simulink model "EsamblajeCohete2_0"  (R2022a)
settings: Solver=VariableStepAuto  StartTime=0.0  StopTime=10.0  RelTol=1e-3
model workspace: external: MATLAB File C:\Users\SEBASTIANDIAZPABON\OneDrive - Universidad Santo Tomás Bucaramanga\USTA\Semillero Cohete\Cohete Matlab 2.0\EsamblajeCohete2_0_DataFile.m (data not in the file)
undefined symbols (not defined in the file or in its folder): smiData, X, Y, Z
libraries: sm_lib x340, simulink x39, nesl_utility x9
(part 4 of 6)

== system EsamblajeCohete2_0/Cohete/x13_INCH_PROPELLER_2_RIGID ==
  ReferenceFrame : sm_lib/Frames and Transforms/Reference Frame
  Solid : sm_lib/Body Elements/File Solid  ExtGeomFileName=13 INCH PROPELLER_Default_sldprt.STEP  UnitType=FromFile  ExtGeomFileUnits=m  StepReaderType=HEX  ExportConvexHullGeometry=off  InertiaType=Custom  Mass=smiData.Solid(1).mass  MassUnits=kg  CenterOfMass=smiData.Solid(1).CoM  CenterOfMassUnits=mm  MomentsOfInertia=smiData.Solid(1).MoI  MomentsOfInertiaUnits=kg*mm^2  ProductsOfInertia=smiData.Solid(1).PoI  ProductsOfInertiaUnits=kg*mm^2  BasedOnType=DensityFromFile  Density=1000  DensityUnits=kg/m^3  DoExposeReferenceFrame=on  SerializedFrames=<Frames/>  GraphicType=FromGeometry  MarkerShape=Sphere  MarkerSize=10  GraphicVisPropType=SimpleVisualProperties  GraphicDiffuseColor=smiData.Solid(1).color  GraphicSpecularColor=[0.5 0.5 0.5 1.0]  GraphicAmbientColor=[0.15 0.15 0.15 1.0]  GraphicEmissiveColor=[0.0 0.0 0.0 1.0]  GraphicShininess=75  GraphicOpacity=smiData.Solid(1).opacity
  Transform : sm_lib/Frames and Transforms/Rigid Transform  TranslationMethod=Cartesian  TranslationStandardOffset=0  TranslationLengthUnit=mm  TranslationStandardAxis=+Z  TranslationCartesianOffset=smiData.RigidTransform(4).translation  TranslationROffset=0  TranslationROffsetUnits=m  TranslationZOffset=0  TranslationZOffsetUnits=m  TranslationThetaOffset=0  TranslationThetaOffsetUnits=deg  RotationMethod=ArbitraryAxis  RotationAngleUnits=rad  RotationStandardAxis=+Z  RotationAngle=smiData.RigidTransform(4).angle  RotationArbitraryAxis=smiData.RigidTransform(4).axis  FollAlignAxisA=+X  BaseAlignAxisA=+Y  FollAlignAxisB=+Y  BaseAlignAxisB=+Z  RotationSequenceAxes=FollowerAxes  RotationSequence=XYX  RotationSequenceAngles=[0 0 0]  RotationSequenceAnglesUnits=deg  RotationMatrix=[1 0 0; 0 1 0; 0 0 1]
  F : PMIOPort  Side=Left
  connections:
  Solid/RConn1 -- ReferenceFrame/RConn1 -- Transform/LConn1
  Transform/RConn1 -- F/RConn1

== system EsamblajeCohete2_0/Cohete/x13_INCH_PROPELLER_3_RIGID ==
  ReferenceFrame : sm_lib/Frames and Transforms/Reference Frame
  Solid : sm_lib/Body Elements/File Solid  ExtGeomFileName=13 INCH PROPELLER_Default_sldprt.STEP  UnitType=FromFile  ExtGeomFileUnits=m  StepReaderType=HEX  ExportConvexHullGeometry=off  InertiaType=Custom  Mass=smiData.Solid(1).mass  MassUnits=kg  CenterOfMass=smiData.Solid(1).CoM  CenterOfMassUnits=mm  MomentsOfInertia=smiData.Solid(1).MoI  MomentsOfInertiaUnits=kg*mm^2  ProductsOfInertia=smiData.Solid(1).PoI  ProductsOfInertiaUnits=kg*mm^2  BasedOnType=DensityFromFile  Density=1000  DensityUnits=kg/m^3  DoExposeReferenceFrame=on  SerializedFrames=<Frames/>  GraphicType=FromGeometry  MarkerShape=Sphere  MarkerSize=10  GraphicVisPropType=SimpleVisualProperties  GraphicDiffuseColor=smiData.Solid(1).color  GraphicSpecularColor=[0.5 0.5 0.5 1.0]  GraphicAmbientColor=[0.15 0.15 0.15 1.0]  GraphicEmissiveColor=[0.0 0.0 0.0 1.0]  GraphicShininess=75  GraphicOpacity=smiData.Solid(1).opacity
  Transform : sm_lib/Frames and Transforms/Rigid Transform  TranslationMethod=Cartesian  TranslationStandardOffset=0  TranslationLengthUnit=mm  TranslationStandardAxis=+Z  TranslationCartesianOffset=smiData.RigidTransform(6).translation  TranslationROffset=0  TranslationROffsetUnits=m  TranslationZOffset=0  TranslationZOffsetUnits=m  TranslationThetaOffset=0  TranslationThetaOffsetUnits=deg  RotationMethod=ArbitraryAxis  RotationAngleUnits=rad  RotationStandardAxis=+Z  RotationAngle=smiData.RigidTransform(6).angle  RotationArbitraryAxis=smiData.RigidTransform(6).axis  FollAlignAxisA=+X  BaseAlignAxisA=+Y  FollAlignAxisB=+Y  BaseAlignAxisB=+Z  RotationSequenceAxes=FollowerAxes  RotationSequence=XYX  RotationSequenceAngles=[0 0 0]  RotationSequenceAnglesUnits=deg  RotationMatrix=[1 0 0; 0 1 0; 0 0 1]
  F : PMIOPort  Side=Left
  connections:
  Solid/RConn1 -- ReferenceFrame/RConn1 -- Transform/LConn1
  Transform/RConn1 -- F/RConn1

== system EsamblajeCohete2_0/Cohete/x13_INCH_PROPELLER_4_RIGID ==
  ReferenceFrame : sm_lib/Frames and Transforms/Reference Frame
  Solid : sm_lib/Body Elements/File Solid  ExtGeomFileName=13 INCH PROPELLER_Default_sldprt.STEP  UnitType=FromFile  ExtGeomFileUnits=m  StepReaderType=HEX  ExportConvexHullGeometry=off  InertiaType=Custom  Mass=smiData.Solid(1).mass  MassUnits=kg  CenterOfMass=smiData.Solid(1).CoM  CenterOfMassUnits=mm  MomentsOfInertia=smiData.Solid(1).MoI  MomentsOfInertiaUnits=kg*mm^2  ProductsOfInertia=smiData.Solid(1).PoI  ProductsOfInertiaUnits=kg*mm^2  BasedOnType=DensityFromFile  Density=1000  DensityUnits=kg/m^3  DoExposeReferenceFrame=on  SerializedFrames=<Frames/>  GraphicType=FromGeometry  MarkerShape=Sphere  MarkerSize=10  GraphicVisPropType=SimpleVisualProperties  GraphicDiffuseColor=smiData.Solid(1).color  GraphicSpecularColor=[0.5 0.5 0.5 1.0]  GraphicAmbientColor=[0.15 0.15 0.15 1.0]  GraphicEmissiveColor=[0.0 0.0 0.0 1.0]  GraphicShininess=75  GraphicOpacity=smiData.Solid(1).opacity
  Transform : sm_lib/Frames and Transforms/Rigid Transform  TranslationMethod=Cartesian  TranslationStandardOffset=0  TranslationLengthUnit=mm  TranslationStandardAxis=+Z  TranslationCartesianOffset=smiData.RigidTransform(8).translation  TranslationROffset=0  TranslationROffsetUnits=m  TranslationZOffset=0  TranslationZOffsetUnits=m  TranslationThetaOffset=0  TranslationThetaOffsetUnits=deg  RotationMethod=ArbitraryAxis  RotationAngleUnits=rad  RotationStandardAxis=+Z  RotationAngle=smiData.RigidTransform(8).angle  RotationArbitraryAxis=smiData.RigidTransform(8).axis  FollAlignAxisA=+X  BaseAlignAxisA=+Y  FollAlignAxisB=+Y  BaseAlignAxisB=+Z  RotationSequenceAxes=FollowerAxes  RotationSequence=XYX  RotationSequenceAngles=[0 0 0]  RotationSequenceAnglesUnits=deg  RotationMatrix=[1 0 0; 0 1 0; 0 0 1]
  F : PMIOPort  Side=Left
  connections:
  Solid/RConn1 -- ReferenceFrame/RConn1 -- Transform/LConn1
  Transform/RConn1 -- F/RConn1

== system EsamblajeCohete2_0/Dinámica /Constantes ==
  Masa : Constant  Value=1.6
  gravedad : Constant  Value=9.81
  ixx : Constant  Value=0.04
  ixx1 : Constant  Value=0.04
  iyy : Constant  Value=0.02
  kd : Constant
  kt : Constant
  longitud : Constant  Value=0.2923
  m : Outport
  g : Outport  Port=2
  Ixx : Outport  Port=3
  Iyy : Outport  Port=4
  Izz : Outport  Port=5
  L : Outport  Port=6
  Κτ : Outport  Port=7
  Kd : Outport  Port=8
  wires:
  Masa/1 -> m/1
  gravedad/1 -> g/1
  ixx/1 -> Ixx/1
  iyy/1 -> Iyy/1
  ixx1/1 -> Izz/1
  longitud/1 -> L/1
  kt/1 -> Κτ/1
  kd/1 -> Kd/1

== system EsamblajeCohete2_0/Dinámica /Torque Yaw ==
  note: $\tau_\psi=\sum_{i=1}^4 \tau_{M i}=K_d \cdot\left(-\omega_1^2+\omega_2^2-\omega_3^2+\omega_4^2\right)$
  ω1 : Inport
  ω2 : Inport  Port=2
  ω3 : Inport  Port=3
  ω4 : Inport  Port=4
  Kd : Inport  Port=5
  Add : Sum  Inputs=-+-+
  Dot Product{,1..7} (8 alike) : DotProduct  OutDataTypeStr=Inherit: Inherit via internal rule
  Tψ : Outport
  wires:
  ω1/1 -> Dot Product/1, Dot Product/2
  Dot Product1/1 -> Add/1
  Dot Product/1 -> Dot Product1/2
  Kd/1 -> Dot Product7/1, Dot Product5/1, Dot Product3/1, Dot Product1/1
  ω2/1 -> Dot Product2/2, Dot Product2/1
  Dot Product2/1 -> Dot Product3/2
  Dot Product3/1 -> Add/2
  ω3/1 -> Dot Product4/2, Dot Product4/1
  Dot Product4/1 -> Dot Product5/2
  Dot Product5/1 -> Add/3
  ω4/1 -> Dot Product6/2, Dot Product6/1
  Dot Product6/1 -> Dot Product7/2
  Dot Product7/1 -> Add/4
  Add/1 -> Tψ/1

== system EsamblajeCohete2_0/Dinámica /Torques Roll y Pitch ==
  note: $\tau_\phi=l \cdot\left(f_4-f_2\right)$
  note: $\tau_\theta=l \cdot\left(f_3-f_1\right)$
  L : Inport
  f1 : Inport  Port=2
  f2 : Inport  Port=3
  f3 : Inport  Port=4
  f4 : Inport  Port=5
  Add : Sum  Inputs=+-
  Add1 : Sum  Inputs=+-
  Product{,1..3} (4 alike) : Product
  Tφ : Outport
  Tθ : Outport  Port=2
  wires:
  f1/1 -> Product/2
  L/1 -> Product1/1, Product3/1, Product2/1, Product/1
  f3/1 -> Product1/2
  Product1/1 -> Add/1
  Product/1 -> Add/2
  Add/1 -> Tθ/1
  f4/1 -> Product2/2
  f2/1 -> Product3/2
  Product2/1 -> Add1/1
  Product3/1 -> Add1/2
  Add1/1 -> Tφ/1

== system EsamblajeCohete2_0/Dinámica /Z'' ==
  note: $\ddot{z}=\frac{f}{m} cos( \phi) cos( \theta)-g$
  f : Inport
  m : Inport  Port=2
  g : Inport  Port=3
  ϕ : Inport  Port=4
  θ : Inport  Port=5
  Add : Sum  Inputs=+-
  Divide : Product  Inputs=*/
  Dot Product1 : DotProduct  OutDataTypeStr=Inherit: Inherit via internal rule
  Integrator : Integrator
  Integrator1 : Integrator
  Product2 : Product
  cos(θ) : simulink/Lookup Tables/Cosine  Formula=cos(2*pi*u)  NumDataPoints=(2^5)+1  OutputWordLength=16  InternalRulePriority=Speed
      settings: SourceProductBaseCode=SL
  cos(ϕ) : simulink/Lookup Tables/Cosine  Formula=cos(2*pi*u)  NumDataPoints=(2^5)+1  OutputWordLength=16  InternalRulePriority=Speed
      settings: SourceProductBaseCode=SL
  Z : Outport
  wires:
  g/1 -> Add/2
  f/1 -> Divide/1
  m/1 -> Divide/2
  Divide/1 -> Product2/1
  Product2/1 -> Add/1
  Integrator1/1 -> Z/1
  Integrator/1 -> Integrator1/1
  Add/1 -> Integrator/1
  θ/1 -> cos(θ)/1
  ϕ/1 -> cos(ϕ)/1
  cos(ϕ)/1 -> Dot Product1/1
  cos(θ)/1 -> Dot Product1/2
  Dot Product1/1 -> Product2/2

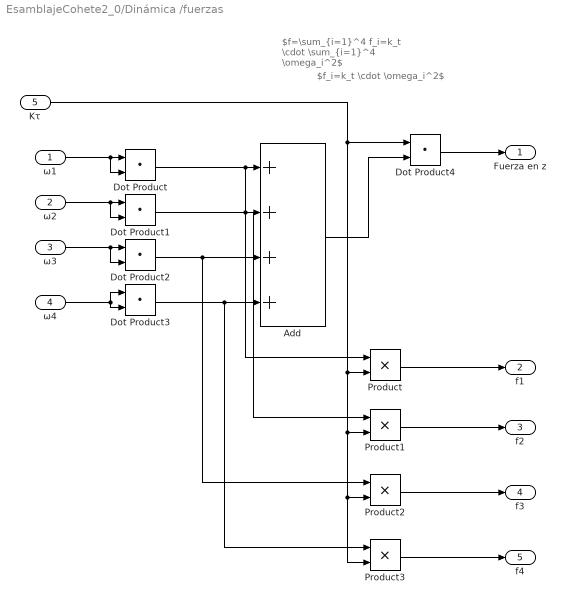
== system EsamblajeCohete2_0/Dinámica /fuerzas ==
  note: $f_i=k_t \cdot \omega_i^2$
  note: $f=\sum_{i=1}^4 f_i=k_t \cdot \sum_{i=1}^4 \omega_i^2$
  ω1 : Inport
  ω2 : Inport  Port=2
  ω3 : Inport  Port=3
  ω4 : Inport  Port=4
  Κτ : Inport  Port=5
  Add : Sum  Inputs=++++
  Dot Product{,1..4} (5 alike) : DotProduct  OutDataTypeStr=Inherit: Inherit via internal rule
  Product{,1..3} (4 alike) : Product
  Fuerza en z : Outport
  f1 : Outport  Port=2
  f2 : Outport  Port=3
  f3 : Outport  Port=4
  f4 : Outport  Port=5
  wires:
  ω1/1 -> Dot Product/2, Dot Product/1
  Dot Product/1 -> Product/1, Add/1
  ω2/1 -> Dot Product1/2, Dot Product1/1
  ω3/1 -> Dot Product2/2, Dot Product2/1
  ω4/1 -> Dot Product3/1, Dot Product3/2
  Dot Product1/1 -> Product1/1, Add/2
  Dot Product2/1 -> Product2/1, Add/3
  Dot Product3/1 -> Product3/1, Add/4
  Dot Product4/1 -> Fuerza en z/1
  Κτ/1 -> Product3/2, Product2/2, Product1/2, Product/2, Dot Product4/1
  Add/1 -> Dot Product4/2
  Product/1 -> f1/1
  Product1/1 -> f2/1
  Product2/1 -> f3/1
  Product3/1 -> f4/1

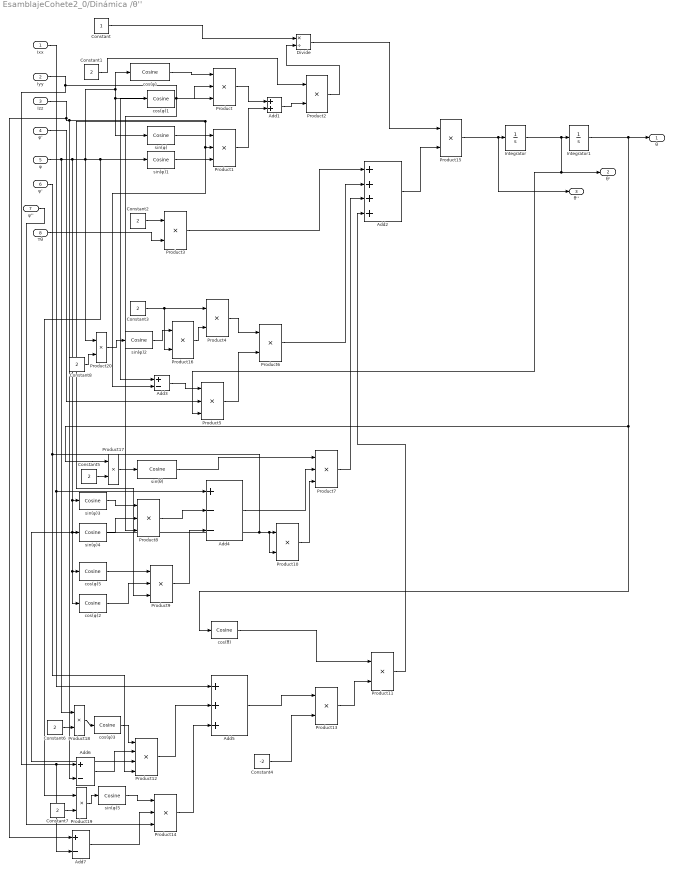
== system EsamblajeCohete2_0/Dinámica /θ'' ==
  Ixx : Inport
  Iyy : Inport  Port=2
  Izz : Inport  Port=3
  φ' : Inport  Port=4
  φ : Inport  Port=5
  ψ' : Inport  Port=6
  ψ'' : Inport  Port=7
  Tθ : Inport  Port=8
  Add1 : Sum
  Add2 : Sum  Inputs=++++
  Add3 : Sum  Inputs=+-
  Add4 : Sum  Inputs=+--
  Add5 : Sum  Inputs=+++
  Add6 : Sum  Inputs=+-
  Add7 : Sum  Inputs=+-
  Constant : Constant
  Constant{1..3,5..8} (7 alike) : Constant  Value=2
  Constant4 : Constant  Value=-2
  Divide : Product  Inputs=*/
  Integrator : Integrator
  Integrator1 : Integrator
  Product{,1,5,7..9,14} (7 alike) : Product  Inputs=3
  Product{2..4,6,10..11,13,15..20} (13 alike) : Product
  Product12 : Product  Inputs=4
  cos(θ) : simulink/Lookup Tables/Cosine  Formula=cos(2*pi*u)  NumDataPoints=(2^5)+1  OutputWordLength=16  InternalRulePriority=Speed
      settings: SourceProductBaseCode=SL
  cos(φ){,1..3,5} (5 alike) : simulink/Lookup Tables/Cosine  Formula=cos(2*pi*u)  NumDataPoints=(2^5)+1  OutputWordLength=16  InternalRulePriority=Speed
      settings: SourceProductBaseCode=SL
  sin(θ) : simulink/Lookup Tables/Cosine  Formula=sin(2*pi*u)  NumDataPoints=(2^5)+1  OutputWordLength=16  InternalRulePriority=Speed
      settings: SourceProductBaseCode=SL
  sin(φ){,1..5} (6 alike) : simulink/Lookup Tables/Cosine  Formula=sin(2*pi*u)  NumDataPoints=(2^5)+1  OutputWordLength=16  InternalRulePriority=Speed
      settings: SourceProductBaseCode=SL
  θ : Outport
  θ' : Outport  Port=2
  θ'' : Outport  Port=3
  wires:
  Constant/1 -> Divide/1
  φ/1 -> Product18/1, cos(φ)2/1, cos(φ)5/1, sin(φ)4/1, sin(φ)3/1, Product20/1, Product19/1, sin(φ)1/1, cos(φ)1/1, sin(φ)/1, cos(φ)/1
  cos(φ)/1 -> Product/1
  cos(φ)1/1 -> Product/2
  Iyy/1 -> Add7/2, Add6/1, Add3/1, Product/3, Product8/3
  sin(φ)/1 -> Product1/1
  sin(φ)1/1 -> Product1/3
  Izz/1 -> Add7/1, Add3/2, Product1/2, Product9/3, Add6/2
  Product/1 -> Add1/1
  Product1/1 -> Add1/2
  Add1/1 -> Product2/2
  Constant1/1 -> Product2/1
  Product2/1 -> Divide/2
  Constant2/1 -> Product3/1
  Tθ/1 -> Product3/2
  Product3/1 -> Add2/1
  Constant3/1 -> Product16/2, Product4/1
  sin(φ)2/1 -> Product16/1
  Add3/1 -> Product5/1
  φ'/1 -> Product5/2
  Product4/1 -> Product6/1
  Product5/1 -> Product6/2
  Product6/1 -> Add2/2
  sin(θ)/1 -> Product7/1
  Ixx/1 -> Add5/1, Add4/1
  sin(φ)4/1 -> Product8/2
  sin(φ)3/1 -> Product8/1
  Product8/1 -> Add4/2
  cos(φ)5/1 -> Product9/1
  cos(φ)2/1 -> Product9/2
  Product9/1 -> Add4/3
  Add4/1 -> Product7/2
  ψ'/1 -> Product12/4, Product12/3, Product10/2, Product10/1
  Product10/1 -> Product7/3
  cos(θ)/1 -> Product11/1
  cos(φ)3/1 -> Product12/1
  Add6/1 -> Product12/2
  Product12/1 -> Add5/2
  Constant4/1 -> Product13/2
  Add5/1 -> Product13/1
  Product13/1 -> Product11/2
  sin(φ)5/1 -> Product14/1
  Add7/1 -> Product14/2
  Product14/1 -> Add5/3
  ψ''/1 -> Product14/3
  Product7/1 -> Add2/3
  Product11/1 -> Add2/4
  Divide/1 -> Product15/1
  Add2/1 -> Product15/2
  Product15/1 -> θ''/1, Integrator/1
  Integrator/1 -> θ'/1, Product5/3, Integrator1/1
  Integrator1/1 -> Product17/1, cos(θ)/1, θ/1
  Product16/1 -> Product4/2
  Product17/1 -> sin(θ)/1
  Constant5/1 -> Product17/2
  Constant6/1 -> Product18/2
  Product18/1 -> cos(φ)3/1
  Constant7/1 -> Product19/2
  Product19/1 -> sin(φ)5/1
  Constant8/1 -> Product20/2
  Product20/1 -> sin(φ)2/1

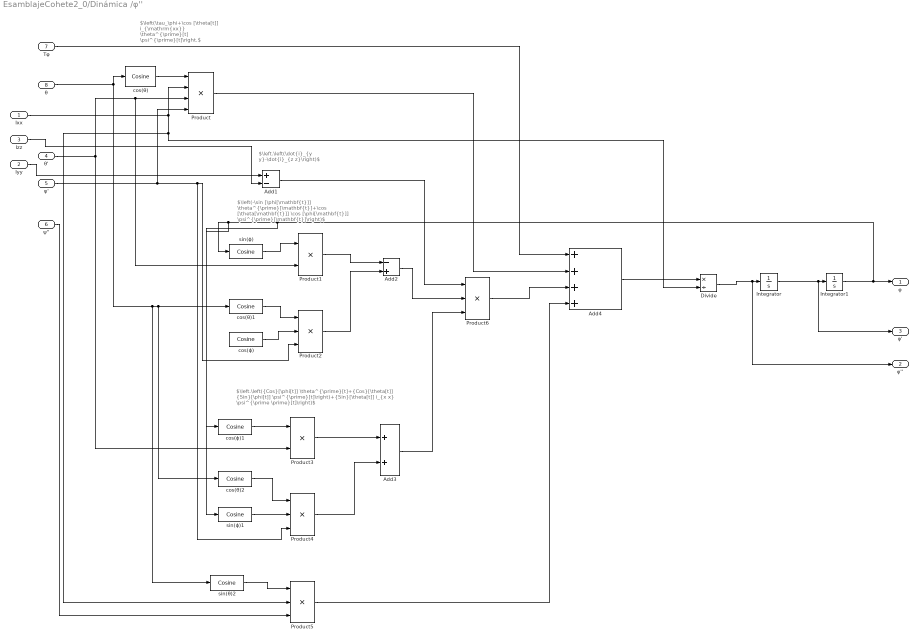
== system EsamblajeCohete2_0/Dinámica /φ'' ==
  note: $\left.\left({Cos}[\phi[t]] \theta^{\prime}[t]+{Cos}[\theta[t]] {Sin}[\phi[t]] \psi^{\prime}[t]\right)+{Sin}[\theta[t]] i_{x x} \psi^{\prime \prime}[t]\right)$
  note: $\left(-\sin [\phi[\mathbf{t}]] \theta^{\prime}[\mathbf{t}]+\cos [\theta[\mathbf{t}]] \cos [\phi[\mathbf{t}]] \psi^{\prime}[\mathbf{t}]\right)$
  note: $\left.\left(\dot{i}_{y y}-\dot{i}_{z z}\right)$
  note: $\left(\tau_\phi+\cos [\theta[t]] i_{\mathrm{xx}} \theta^{\prime}[t] \psi^{\prime}[t]\right.$
  Ixx : Inport
  Iyy : Inport  Port=2
  Izz : Inport  Port=3
  θ' : Inport  Port=4
  ψ' : Inport  Port=5
  ψ'' : Inport  Port=6
  Tφ : Inport  Port=7
  θ : Inport  Port=8
  Add1 : Sum  Inputs=+-
  Add2 : Sum  Inputs=-+
  Add3 : Sum
  Add4 : Sum  Inputs=++++
  Divide : Product  Inputs=*/
  Integrator : Integrator
  Integrator1 : Integrator
  Product : Product  Inputs=4
  Product1 : Product
  Product{2,4..6} (4 alike) : Product  Inputs=3
  Product3 : Product
  cos(θ) : simulink/Lookup Tables/Cosine  Formula=cos(2*pi*u)  NumDataPoints=(2^5)+1  OutputWordLength=16  InternalRulePriority=Speed
      settings: SourceProductBaseCode=SL
  cos(θ)1 : simulink/Lookup Tables/Cosine  Formula=cos(2*pi*u)  NumDataPoints=(2^5)+1  OutputWordLength=16  InternalRulePriority=Speed
      settings: SourceProductBaseCode=SL
  cos(θ)2 : simulink/Lookup Tables/Cosine  Formula=cos(2*pi*u)  NumDataPoints=(2^5)+1  OutputWordLength=16  InternalRulePriority=Speed
      settings: SourceProductBaseCode=SL
  cos(ϕ) : simulink/Lookup Tables/Cosine  Formula=cos(2*pi*u)  NumDataPoints=(2^5)+1  OutputWordLength=16  InternalRulePriority=Speed
      settings: SourceProductBaseCode=SL
  cos(ϕ)1 : simulink/Lookup Tables/Cosine  Formula=cos(2*pi*u)  NumDataPoints=(2^5)+1  OutputWordLength=16  InternalRulePriority=Speed
      settings: SourceProductBaseCode=SL
  sin(θ)2 : simulink/Lookup Tables/Cosine  Formula=sin(2*pi*u)  NumDataPoints=(2^5)+1  OutputWordLength=16  InternalRulePriority=Speed
      settings: SourceProductBaseCode=SL
  sin(ϕ) : simulink/Lookup Tables/Cosine  Formula=sin(2*pi*u)  NumDataPoints=(2^5)+1  OutputWordLength=16  InternalRulePriority=Speed
      settings: SourceProductBaseCode=SL
  sin(ϕ)1 : simulink/Lookup Tables/Cosine  Formula=sin(2*pi*u)  NumDataPoints=(2^5)+1  OutputWordLength=16  InternalRulePriority=Speed
      settings: SourceProductBaseCode=SL
  φ : Outport
  φ'' : Outport  Port=2
  φ' : Outport  Port=3
  wires:
  θ/1 -> cos(θ)1/1, cos(θ)2/1, sin(θ)2/1, cos(θ)/1
  cos(θ)/1 -> Product/1
  Ixx/1 -> Product/2, Product5/2, Divide/2
  θ'/1 -> Product3/2, Product/3, Product1/2
  ψ'/1 -> Product2/3, Product4/3, Product/4
  Iyy/1 -> Add1/1
  Izz/1 -> Add1/2
  sin(ϕ)/1 -> Product1/1
  Product1/1 -> Add2/1
  cos(θ)1/1 -> Product2/1
  cos(ϕ)/1 -> Product2/2
  Product2/1 -> Add2/2
  cos(ϕ)1/1 -> Product3/1
  cos(θ)2/1 -> Product4/1
  sin(ϕ)1/1 -> Product4/2
  sin(θ)2/1 -> Product5/1
  ψ''/1 -> Product5/3
  Product3/1 -> Add3/1
  Product4/1 -> Add3/2
  Add1/1 -> Product6/1
  Add2/1 -> Product6/2
  Add3/1 -> Product6/3
  Tφ/1 -> Add4/1
  Product/1 -> Add4/2
  Product6/1 -> Add4/3
  Product5/1 -> Add4/4
  Add4/1 -> Divide/1
  Divide/1 -> φ''/1, Integrator/1
  Integrator/1 -> φ'/1, Integrator1/1
  Integrator1/1 -> sin(ϕ)1/1, cos(ϕ)1/1, sin(ϕ)/1, φ/1

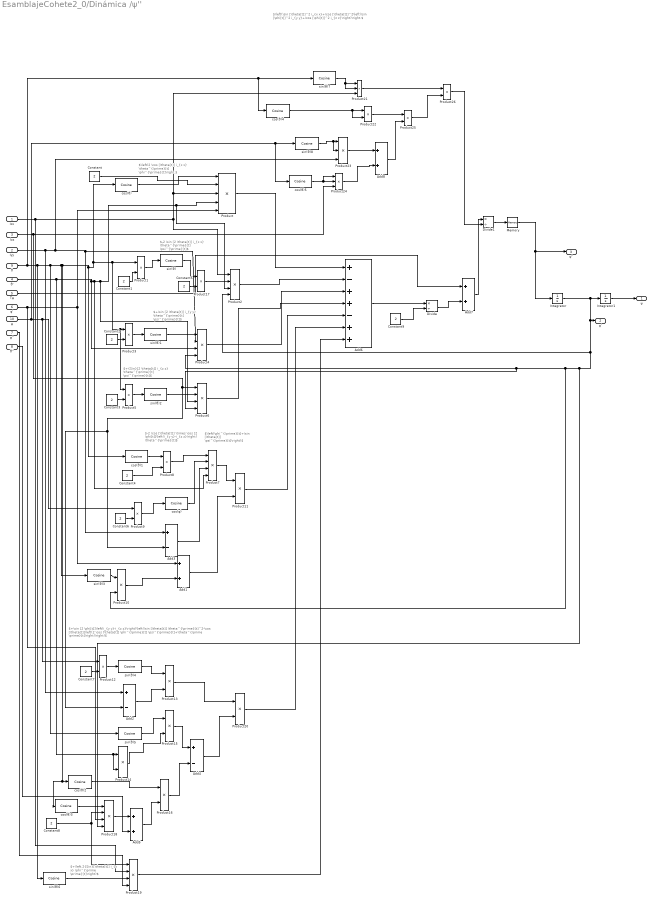
== system EsamblajeCohete2_0/Dinámica /ψ'' ==
  note: $\left(\sin [\theta[t]]^2 i_{x x}+\cos [\theta[t]]^2\left(\sin [\phi[t]]^2 i_{y y}+\cos [\phi[t]]^2 i_{z z}\right)\right.$
  note: $+\left.2{Sin}[\theta[t]] i_{x x} \phi^{\prime \prime}[t]\right)$
  note: $+\sin [2 \phi[t]]\left(i_{y y}-i_{z z}\right)\left(\sin [\theta[t]] \theta^{\prime}[t]^2-\cos [\theta[t]]\left(2 \cos [\theta[t]] \phi^{\prime}[t] \psi^{\prime}[t]+\theta^{\prime \prime}[t]\right)\right)$
  note: $\left(\phi^{\prime}[t]+\sin [\theta[t]] \psi^{\prime}[t]\right)$
  note: $-2 \cos [\theta[t]] \times \cos [2 \phi[t]]\left(i_{y y}-i_{z z}\right) \theta^{\prime}[t]$
  note: $+{Sin}[2 \theta[t]] i_{z z} \theta^{\prime}[t] \psi^{\prime}[t]$
  note: $+\sin [2 \theta[t]] i_{y y} \theta^{\prime}[t] \psi^{\prime}[t]$
  note: $-2 \sin [2 \theta[t]] i_{x x} \theta^{\prime}[t] \psi^{\prime}[t]$
  note: $\left(2 \cos [\theta[t]] i_{x x} \theta^{\prime}[t] \phi^{\prime}[t]\right.$
  Ixx : Inport
  Iyy : Inport  Port=2
  Izz : Inport  Port=3
  θ' : Inport  Port=4
  Tψ : Inport  Port=5
  φ' : Inport  Port=6
  φ'' : Inport  Port=7
  θ'' : Inport  Port=8
  θ : Inport  Port=9
  φ : Inport  Port=10
  Add{1,5,7..8} (4 alike) : Sum
  Add2 : Sum  Inputs=+-
  Add3 : Sum  Inputs=+-
  Add4 : Sum  Inputs=+-
  Add6 : Sum  Inputs=+-++-++
  Constant{,1..9} (10 alike) : Constant  Value=2
  Divide : Product  Inputs=*/
  Divide1 : Product  Inputs=*/
  Integrator : Integrator
  Integrator1 : Integrator
  Memory : Memory
  Product : Product  Inputs=5
  Product{1,3,5,8..17,20,22,25..26} (17 alike) : Product
  Product{2,4,6..7,18..19} (6 alike) : Product  Inputs=4
  Product21 : Product  Inputs=3
  Product23 : Product  Inputs=3
  Product24 : Product  Inputs=3
  cos(θ){,1..5} (6 alike) : simulink/Lookup Tables/Cosine  Formula=cos(2*pi*u)  NumDataPoints=(2^5)+1  OutputWordLength=16  InternalRulePriority=Speed
      settings: SourceProductBaseCode=SL
  cos(φ) : simulink/Lookup Tables/Cosine  Formula=cos(2*pi*u)  NumDataPoints=(2^5)+1  OutputWordLength=16  InternalRulePriority=Speed
      settings: SourceProductBaseCode=SL
  sin(θ){,1..8} (9 alike) : simulink/Lookup Tables/Cosine  Formula=sin(2*pi*u)  NumDataPoints=(2^5)+1  OutputWordLength=16  InternalRulePriority=Speed
      settings: SourceProductBaseCode=SL
  ψ : Outport
  ψ' : Outport  Port=2
  ψ'' : Outport  Port=3
  wires:
  θ/1 -> sin(θ)7/1, cos(θ)4/1, sin(θ)5/1, cos(θ)3/1, cos(θ)2/1, cos(θ)1/1, Product1/1, Product5/1, Product3/1, cos(θ)/1, sin(θ)3/1, sin(θ)6/1
  cos(θ)/1 -> Product/1
  Constant/1 -> Product/2
  Ixx/1 -> Product19/2, Product21/3, Product/3, Product2/1
  θ'/1 -> Product4/3, Product7/4, Product6/3, Product2/3, Product/4, Product14/2, Product14/1
  φ'/1 -> Product18/3, Add1/1, Product/5
  Constant5/1 -> Product17/2
  sin(θ)/1 -> Product17/1
  Constant1/1 -> Product1/2
  Product1/1 -> sin(θ)/1
  Product17/1 -> Product2/2
  Constant2/1 -> Product3/2
  Product3/1 -> sin(θ)1/1
  sin(θ)1/1 -> Product4/1
  Iyy/1 -> Add2/1, Product23/3, Add3/1, Product4/2
  Product5/1 -> sin(θ)2/1
  Constant3/1 -> Product5/2
  sin(θ)2/1 -> Product6/2
  Izz/1 -> Product24/3, Add3/2, Add2/2, Product6/1
  cos(θ)1/1 -> Product8/1
  Constant4/1 -> Product8/2
  Product8/1 -> Product7/1
  Product9/1 -> cos(φ)/1
  Constant6/1 -> Product9/2
  φ/1 -> cos(θ)5/1, sin(θ)8/1, Product12/1, Product9/1
  cos(φ)/1 -> Product7/2
  Add3/1 -> Product7/3
  sin(θ)3/1 -> Product10/1
  Product10/1 -> Add1/2
  Product7/1 -> Product11/1
  Add1/1 -> Product11/2
  Constant7/1 -> Product12/2
  Product12/1 -> sin(θ)4/1
  sin(θ)4/1 -> Product13/1
  Add2/1 -> Product13/2
  sin(θ)5/1 -> Product15/1
  Product14/1 -> Product15/2
  Product15/1 -> Add4/1
  cos(θ)2/1 -> Product16/1
  Product16/1 -> Add4/2
  cos(θ)3/1 -> Product18/1
  Constant8/1 -> Product19/1, Product18/2
  Product18/1 -> Add5/1
  Add5/1 -> Product16/2
  θ''/1 -> Add5/2
  sin(θ)6/1 -> Product19/3
  φ''/1 -> Product19/4
  Product/1 -> Add6/1
  Product13/1 -> Product20/1
  Add4/1 -> Product20/2
  Product2/1 -> Add6/2
  Product4/1 -> Add6/3
  Product6/1 -> Add6/4
  Product11/1 -> Add6/5
  Product20/1 -> Add6/6
  Product19/1 -> Add6/7
  Add6/1 -> Divide/1
  Constant9/1 -> Divide/2
  Divide/1 -> Add7/2
  Tψ/1 -> Add7/1
  Add7/1 -> Divide1/1
  Divide1/1 -> Memory/1
  Integrator/1 -> Product2/4, Product18/4, Product10/2, Product6/4, Product4/4, ψ'/1, Integrator1/1
  Integrator1/1 -> ψ/1
  sin(θ)7/1 -> Product21/2, Product21/1
  cos(θ)4/1 -> Product22/2, Product22/1
  sin(θ)8/1 -> Product23/2, Product23/1
  cos(θ)5/1 -> Product24/2, Product24/1
  Product23/1 -> Add8/1
  Product24/1 -> Add8/2
  Product22/1 -> Product25/1
  Add8/1 -> Product25/2
  Product21/1 -> Product26/1
  Product25/1 -> Product26/2
  Product26/1 -> Divide1/2
  Memory/1 -> Integrator/1, ψ''/1

== system EsamblajeCohete2_0/Cohete/Assembly_1_RIGID/Drive_Shaft_1_RIGID ==
  ReferenceFrame : sm_lib/Frames and Transforms/Reference Frame
  Solid : sm_lib/Body Elements/File Solid  ExtGeomFileName=Drive Shaft_Default_sldprt.STEP  UnitType=FromFile  ExtGeomFileUnits=m  StepReaderType=HEX  ExportConvexHullGeometry=off  InertiaType=Custom  Mass=smiData.Solid(7).mass  MassUnits=kg  CenterOfMass=smiData.Solid(7).CoM  CenterOfMassUnits=mm  MomentsOfInertia=smiData.Solid(7).MoI  MomentsOfInertiaUnits=kg*mm^2  ProductsOfInertia=smiData.Solid(7).PoI  ProductsOfInertiaUnits=kg*mm^2  BasedOnType=DensityFromFile  Density=1000  DensityUnits=kg/m^3  DoExposeReferenceFrame=on  SerializedFrames=<Frames/>  GraphicType=FromGeometry  MarkerShape=Sphere  MarkerSize=10  GraphicVisPropType=SimpleVisualProperties  GraphicDiffuseColor=smiData.Solid(7).color  GraphicSpecularColor=[0.5 0.5 0.5 1.0]  GraphicAmbientColor=[0.15 0.15 0.15 1.0]  GraphicEmissiveColor=[0.0 0.0 0.0 1.0]  GraphicShininess=75  GraphicOpacity=smiData.Solid(7).opacity
  F : PMIOPort  Side=Left
  connections:
  Solid/RConn1 -- ReferenceFrame/RConn1 -- F/RConn1

== system EsamblajeCohete2_0/Cohete/Assembly_1_RIGID/Electrical_Windings_1_RIGID ==
  ReferenceFrame : sm_lib/Frames and Transforms/Reference Frame
  Solid : sm_lib/Body Elements/File Solid  ExtGeomFileName=Electrical Windings_Default_sldprt.STEP  UnitType=FromFile  ExtGeomFileUnits=m  StepReaderType=HEX  ExportConvexHullGeometry=off  InertiaType=Custom  Mass=smiData.Solid(6).mass  MassUnits=kg  CenterOfMass=smiData.Solid(6).CoM  CenterOfMassUnits=mm  MomentsOfInertia=smiData.Solid(6).MoI  MomentsOfInertiaUnits=kg*mm^2  ProductsOfInertia=smiData.Solid(6).PoI  ProductsOfInertiaUnits=kg*mm^2  BasedOnType=DensityFromFile  Density=1000  DensityUnits=kg/m^3  DoExposeReferenceFrame=on  SerializedFrames=<Frames/>  GraphicType=FromGeometry  MarkerShape=Sphere  MarkerSize=10  GraphicVisPropType=SimpleVisualProperties  GraphicDiffuseColor=smiData.Solid(6).color  GraphicSpecularColor=[0.5 0.5 0.5 1.0]  GraphicAmbientColor=[0.15 0.15 0.15 1.0]  GraphicEmissiveColor=[0.0 0.0 0.0 1.0]  GraphicShininess=75  GraphicOpacity=smiData.Solid(6).opacity
  F : PMIOPort  Side=Left
  connections:
  Solid/RConn1 -- ReferenceFrame/RConn1 -- F/RConn1

== system EsamblajeCohete2_0/Cohete/Assembly_1_RIGID/Magnet_10_RIGID ==
  ReferenceFrame : sm_lib/Frames and Transforms/Reference Frame
  Solid : sm_lib/Body Elements/File Solid  ExtGeomFileName=Magnet_Default_sldprt.STEP  UnitType=FromFile  ExtGeomFileUnits=m  StepReaderType=HEX  ExportConvexHullGeometry=off  InertiaType=Custom  Mass=smiData.Solid(5).mass  MassUnits=kg  CenterOfMass=smiData.Solid(5).CoM  CenterOfMassUnits=mm  MomentsOfInertia=smiData.Solid(5).MoI  MomentsOfInertiaUnits=kg*mm^2  ProductsOfInertia=smiData.Solid(5).PoI  ProductsOfInertiaUnits=kg*mm^2  BasedOnType=DensityFromFile  Density=1000  DensityUnits=kg/m^3  DoExposeReferenceFrame=on  SerializedFrames=<Frames/>  GraphicType=FromGeometry  MarkerShape=Sphere  MarkerSize=10  GraphicVisPropType=SimpleVisualProperties  GraphicDiffuseColor=smiData.Solid(5).color  GraphicSpecularColor=[0.5 0.5 0.5 1.0]  GraphicAmbientColor=[0.15 0.15 0.15 1.0]  GraphicEmissiveColor=[0.0 0.0 0.0 1.0]  GraphicShininess=75  GraphicOpacity=smiData.Solid(5).opacity
  F : PMIOPort  Side=Left
  connections:
  Solid/RConn1 -- ReferenceFrame/RConn1 -- F/RConn1

== system EsamblajeCohete2_0/Cohete/Assembly_1_RIGID/Magnet_11_RIGID ==
  ReferenceFrame : sm_lib/Frames and Transforms/Reference Frame
  Solid : sm_lib/Body Elements/File Solid  ExtGeomFileName=Magnet_Default_sldprt.STEP  UnitType=FromFile  ExtGeomFileUnits=m  StepReaderType=HEX  ExportConvexHullGeometry=off  InertiaType=Custom  Mass=smiData.Solid(5).mass  MassUnits=kg  CenterOfMass=smiData.Solid(5).CoM  CenterOfMassUnits=mm  MomentsOfInertia=smiData.Solid(5).MoI  MomentsOfInertiaUnits=kg*mm^2  ProductsOfInertia=smiData.Solid(5).PoI  ProductsOfInertiaUnits=kg*mm^2  BasedOnType=DensityFromFile  Density=1000  DensityUnits=kg/m^3  DoExposeReferenceFrame=on  SerializedFrames=<Frames/>  GraphicType=FromGeometry  MarkerShape=Sphere  MarkerSize=10  GraphicVisPropType=SimpleVisualProperties  GraphicDiffuseColor=smiData.Solid(5).color  GraphicSpecularColor=[0.5 0.5 0.5 1.0]  GraphicAmbientColor=[0.15 0.15 0.15 1.0]  GraphicEmissiveColor=[0.0 0.0 0.0 1.0]  GraphicShininess=75  GraphicOpacity=smiData.Solid(5).opacity
  F : PMIOPort  Side=Left
  connections:
  Solid/RConn1 -- ReferenceFrame/RConn1 -- F/RConn1

== system EsamblajeCohete2_0/Cohete/Assembly_1_RIGID/Magnet_12_RIGID ==
  ReferenceFrame : sm_lib/Frames and Transforms/Reference Frame
  Solid : sm_lib/Body Elements/File Solid  ExtGeomFileName=Magnet_Default_sldprt.STEP  UnitType=FromFile  ExtGeomFileUnits=m  StepReaderType=HEX  ExportConvexHullGeometry=off  InertiaType=Custom  Mass=smiData.Solid(5).mass  MassUnits=kg  CenterOfMass=smiData.Solid(5).CoM  CenterOfMassUnits=mm  MomentsOfInertia=smiData.Solid(5).MoI  MomentsOfInertiaUnits=kg*mm^2  ProductsOfInertia=smiData.Solid(5).PoI  ProductsOfInertiaUnits=kg*mm^2  BasedOnType=DensityFromFile  Density=1000  DensityUnits=kg/m^3  DoExposeReferenceFrame=on  SerializedFrames=<Frames/>  GraphicType=FromGeometry  MarkerShape=Sphere  MarkerSize=10  GraphicVisPropType=SimpleVisualProperties  GraphicDiffuseColor=smiData.Solid(5).color  GraphicSpecularColor=[0.5 0.5 0.5 1.0]  GraphicAmbientColor=[0.15 0.15 0.15 1.0]  GraphicEmissiveColor=[0.0 0.0 0.0 1.0]  GraphicShininess=75  GraphicOpacity=smiData.Solid(5).opacity
  F : PMIOPort  Side=Left
  connections:
  Solid/RConn1 -- ReferenceFrame/RConn1 -- F/RConn1

== system EsamblajeCohete2_0/Cohete/Assembly_1_RIGID/Magnet_13_RIGID ==
  ReferenceFrame : sm_lib/Frames and Transforms/Reference Frame
  Solid : sm_lib/Body Elements/File Solid  ExtGeomFileName=Magnet_Default_sldprt.STEP  UnitType=FromFile  ExtGeomFileUnits=m  StepReaderType=HEX  ExportConvexHullGeometry=off  InertiaType=Custom  Mass=smiData.Solid(5).mass  MassUnits=kg  CenterOfMass=smiData.Solid(5).CoM  CenterOfMassUnits=mm  MomentsOfInertia=smiData.Solid(5).MoI  MomentsOfInertiaUnits=kg*mm^2  ProductsOfInertia=smiData.Solid(5).PoI  ProductsOfInertiaUnits=kg*mm^2  BasedOnType=DensityFromFile  Density=1000  DensityUnits=kg/m^3  DoExposeReferenceFrame=on  SerializedFrames=<Frames/>  GraphicType=FromGeometry  MarkerShape=Sphere  MarkerSize=10  GraphicVisPropType=SimpleVisualProperties  GraphicDiffuseColor=smiData.Solid(5).color  GraphicSpecularColor=[0.5 0.5 0.5 1.0]  GraphicAmbientColor=[0.15 0.15 0.15 1.0]  GraphicEmissiveColor=[0.0 0.0 0.0 1.0]  GraphicShininess=75  GraphicOpacity=smiData.Solid(5).opacity
  F : PMIOPort  Side=Left
  connections:
  Solid/RConn1 -- ReferenceFrame/RConn1 -- F/RConn1

== system EsamblajeCohete2_0/Cohete/Assembly_1_RIGID/Magnet_14_RIGID ==
  ReferenceFrame : sm_lib/Frames and Transforms/Reference Frame
  Solid : sm_lib/Body Elements/File Solid  ExtGeomFileName=Magnet_Default_sldprt.STEP  UnitType=FromFile  ExtGeomFileUnits=m  StepReaderType=HEX  ExportConvexHullGeometry=off  InertiaType=Custom  Mass=smiData.Solid(5).mass  MassUnits=kg  CenterOfMass=smiData.Solid(5).CoM  CenterOfMassUnits=mm  MomentsOfInertia=smiData.Solid(5).MoI  MomentsOfInertiaUnits=kg*mm^2  ProductsOfInertia=smiData.Solid(5).PoI  ProductsOfInertiaUnits=kg*mm^2  BasedOnType=DensityFromFile  Density=1000  DensityUnits=kg/m^3  DoExposeReferenceFrame=on  SerializedFrames=<Frames/>  GraphicType=FromGeometry  MarkerShape=Sphere  MarkerSize=10  GraphicVisPropType=SimpleVisualProperties  GraphicDiffuseColor=smiData.Solid(5).color  GraphicSpecularColor=[0.5 0.5 0.5 1.0]  GraphicAmbientColor=[0.15 0.15 0.15 1.0]  GraphicEmissiveColor=[0.0 0.0 0.0 1.0]  GraphicShininess=75  GraphicOpacity=smiData.Solid(5).opacity
  F : PMIOPort  Side=Left
  connections:
  Solid/RConn1 -- ReferenceFrame/RConn1 -- F/RConn1

== system EsamblajeCohete2_0/Cohete/Assembly_1_RIGID/Magnet_1_RIGID ==
  ReferenceFrame : sm_lib/Frames and Transforms/Reference Frame
  Solid : sm_lib/Body Elements/File Solid  ExtGeomFileName=Magnet_Default_sldprt.STEP  UnitType=FromFile  ExtGeomFileUnits=m  StepReaderType=HEX  ExportConvexHullGeometry=off  InertiaType=Custom  Mass=smiData.Solid(5).mass  MassUnits=kg  CenterOfMass=smiData.Solid(5).CoM  CenterOfMassUnits=mm  MomentsOfInertia=smiData.Solid(5).MoI  MomentsOfInertiaUnits=kg*mm^2  ProductsOfInertia=smiData.Solid(5).PoI  ProductsOfInertiaUnits=kg*mm^2  BasedOnType=DensityFromFile  Density=1000  DensityUnits=kg/m^3  DoExposeReferenceFrame=on  SerializedFrames=<Frames/>  GraphicType=FromGeometry  MarkerShape=Sphere  MarkerSize=10  GraphicVisPropType=SimpleVisualProperties  GraphicDiffuseColor=smiData.Solid(5).color  GraphicSpecularColor=[0.5 0.5 0.5 1.0]  GraphicAmbientColor=[0.15 0.15 0.15 1.0]  GraphicEmissiveColor=[0.0 0.0 0.0 1.0]  GraphicShininess=75  GraphicOpacity=smiData.Solid(5).opacity
  F : PMIOPort  Side=Left
  connections:
  Solid/RConn1 -- ReferenceFrame/RConn1 -- F/RConn1

== system EsamblajeCohete2_0/Cohete/Assembly_1_RIGID/Magnet_2_RIGID ==
  ReferenceFrame : sm_lib/Frames and Transforms/Reference Frame
  Solid : sm_lib/Body Elements/File Solid  ExtGeomFileName=Magnet_Default_sldprt.STEP  UnitType=FromFile  ExtGeomFileUnits=m  StepReaderType=HEX  ExportConvexHullGeometry=off  InertiaType=Custom  Mass=smiData.Solid(5).mass  MassUnits=kg  CenterOfMass=smiData.Solid(5).CoM  CenterOfMassUnits=mm  MomentsOfInertia=smiData.Solid(5).MoI  MomentsOfInertiaUnits=kg*mm^2  ProductsOfInertia=smiData.Solid(5).PoI  ProductsOfInertiaUnits=kg*mm^2  BasedOnType=DensityFromFile  Density=1000  DensityUnits=kg/m^3  DoExposeReferenceFrame=on  SerializedFrames=<Frames/>  GraphicType=FromGeometry  MarkerShape=Sphere  MarkerSize=10  GraphicVisPropType=SimpleVisualProperties  GraphicDiffuseColor=smiData.Solid(5).color  GraphicSpecularColor=[0.5 0.5 0.5 1.0]  GraphicAmbientColor=[0.15 0.15 0.15 1.0]  GraphicEmissiveColor=[0.0 0.0 0.0 1.0]  GraphicShininess=75  GraphicOpacity=smiData.Solid(5).opacity
  F : PMIOPort  Side=Left
  connections:
  Solid/RConn1 -- ReferenceFrame/RConn1 -- F/RConn1

== system EsamblajeCohete2_0/Cohete/Assembly_1_RIGID/Magnet_3_RIGID ==
  ReferenceFrame : sm_lib/Frames and Transforms/Reference Frame
  Solid : sm_lib/Body Elements/File Solid  ExtGeomFileName=Magnet_Default_sldprt.STEP  UnitType=FromFile  ExtGeomFileUnits=m  StepReaderType=HEX  ExportConvexHullGeometry=off  InertiaType=Custom  Mass=smiData.Solid(5).mass  MassUnits=kg  CenterOfMass=smiData.Solid(5).CoM  CenterOfMassUnits=mm  MomentsOfInertia=smiData.Solid(5).MoI  MomentsOfInertiaUnits=kg*mm^2  ProductsOfInertia=smiData.Solid(5).PoI  ProductsOfInertiaUnits=kg*mm^2  BasedOnType=DensityFromFile  Density=1000  DensityUnits=kg/m^3  DoExposeReferenceFrame=on  SerializedFrames=<Frames/>  GraphicType=FromGeometry  MarkerShape=Sphere  MarkerSize=10  GraphicVisPropType=SimpleVisualProperties  GraphicDiffuseColor=smiData.Solid(5).color  GraphicSpecularColor=[0.5 0.5 0.5 1.0]  GraphicAmbientColor=[0.15 0.15 0.15 1.0]  GraphicEmissiveColor=[0.0 0.0 0.0 1.0]  GraphicShininess=75  GraphicOpacity=smiData.Solid(5).opacity
  F : PMIOPort  Side=Left
  connections:
  Solid/RConn1 -- ReferenceFrame/RConn1 -- F/RConn1

== system EsamblajeCohete2_0/Cohete/Assembly_1_RIGID/Magnet_4_RIGID ==
  ReferenceFrame : sm_lib/Frames and Transforms/Reference Frame
  Solid : sm_lib/Body Elements/File Solid  ExtGeomFileName=Magnet_Default_sldprt.STEP  UnitType=FromFile  ExtGeomFileUnits=m  StepReaderType=HEX  ExportConvexHullGeometry=off  InertiaType=Custom  Mass=smiData.Solid(5).mass  MassUnits=kg  CenterOfMass=smiData.Solid(5).CoM  CenterOfMassUnits=mm  MomentsOfInertia=smiData.Solid(5).MoI  MomentsOfInertiaUnits=kg*mm^2  ProductsOfInertia=smiData.Solid(5).PoI  ProductsOfInertiaUnits=kg*mm^2  BasedOnType=DensityFromFile  Density=1000  DensityUnits=kg/m^3  DoExposeReferenceFrame=on  SerializedFrames=<Frames/>  GraphicType=FromGeometry  MarkerShape=Sphere  MarkerSize=10  GraphicVisPropType=SimpleVisualProperties  GraphicDiffuseColor=smiData.Solid(5).color  GraphicSpecularColor=[0.5 0.5 0.5 1.0]  GraphicAmbientColor=[0.15 0.15 0.15 1.0]  GraphicEmissiveColor=[0.0 0.0 0.0 1.0]  GraphicShininess=75  GraphicOpacity=smiData.Solid(5).opacity
  F : PMIOPort  Side=Left
  connections:
  Solid/RConn1 -- ReferenceFrame/RConn1 -- F/RConn1

== system EsamblajeCohete2_0/Cohete/Assembly_1_RIGID/Magnet_5_RIGID ==
  ReferenceFrame : sm_lib/Frames and Transforms/Reference Frame
  Solid : sm_lib/Body Elements/File Solid  ExtGeomFileName=Magnet_Default_sldprt.STEP  UnitType=FromFile  ExtGeomFileUnits=m  StepReaderType=HEX  ExportConvexHullGeometry=off  InertiaType=Custom  Mass=smiData.Solid(5).mass  MassUnits=kg  CenterOfMass=smiData.Solid(5).CoM  CenterOfMassUnits=mm  MomentsOfInertia=smiData.Solid(5).MoI  MomentsOfInertiaUnits=kg*mm^2  ProductsOfInertia=smiData.Solid(5).PoI  ProductsOfInertiaUnits=kg*mm^2  BasedOnType=DensityFromFile  Density=1000  DensityUnits=kg/m^3  DoExposeReferenceFrame=on  SerializedFrames=<Frames/>  GraphicType=FromGeometry  MarkerShape=Sphere  MarkerSize=10  GraphicVisPropType=SimpleVisualProperties  GraphicDiffuseColor=smiData.Solid(5).color  GraphicSpecularColor=[0.5 0.5 0.5 1.0]  GraphicAmbientColor=[0.15 0.15 0.15 1.0]  GraphicEmissiveColor=[0.0 0.0 0.0 1.0]  GraphicShininess=75  GraphicOpacity=smiData.Solid(5).opacity
  F : PMIOPort  Side=Left
  connections:
  Solid/RConn1 -- ReferenceFrame/RConn1 -- F/RConn1

== system EsamblajeCohete2_0/Cohete/Assembly_1_RIGID/Magnet_6_RIGID ==
  ReferenceFrame : sm_lib/Frames and Transforms/Reference Frame
  Solid : sm_lib/Body Elements/File Solid  ExtGeomFileName=Magnet_Default_sldprt.STEP  UnitType=FromFile  ExtGeomFileUnits=m  StepReaderType=HEX  ExportConvexHullGeometry=off  InertiaType=Custom  Mass=smiData.Solid(5).mass  MassUnits=kg  CenterOfMass=smiData.Solid(5).CoM  CenterOfMassUnits=mm  MomentsOfInertia=smiData.Solid(5).MoI  MomentsOfInertiaUnits=kg*mm^2  ProductsOfInertia=smiData.Solid(5).PoI  ProductsOfInertiaUnits=kg*mm^2  BasedOnType=DensityFromFile  Density=1000  DensityUnits=kg/m^3  DoExposeReferenceFrame=on  SerializedFrames=<Frames/>  GraphicType=FromGeometry  MarkerShape=Sphere  MarkerSize=10  GraphicVisPropType=SimpleVisualProperties  GraphicDiffuseColor=smiData.Solid(5).color  GraphicSpecularColor=[0.5 0.5 0.5 1.0]  GraphicAmbientColor=[0.15 0.15 0.15 1.0]  GraphicEmissiveColor=[0.0 0.0 0.0 1.0]  GraphicShininess=75  GraphicOpacity=smiData.Solid(5).opacity
  F : PMIOPort  Side=Left
  connections:
  Solid/RConn1 -- ReferenceFrame/RConn1 -- F/RConn1

== system EsamblajeCohete2_0/Cohete/Assembly_1_RIGID/Magnet_7_RIGID ==
  ReferenceFrame : sm_lib/Frames and Transforms/Reference Frame
  Solid : sm_lib/Body Elements/File Solid  ExtGeomFileName=Magnet_Default_sldprt.STEP  UnitType=FromFile  ExtGeomFileUnits=m  StepReaderType=HEX  ExportConvexHullGeometry=off  InertiaType=Custom  Mass=smiData.Solid(5).mass  MassUnits=kg  CenterOfMass=smiData.Solid(5).CoM  CenterOfMassUnits=mm  MomentsOfInertia=smiData.Solid(5).MoI  MomentsOfInertiaUnits=kg*mm^2  ProductsOfInertia=smiData.Solid(5).PoI  ProductsOfInertiaUnits=kg*mm^2  BasedOnType=DensityFromFile  Density=1000  DensityUnits=kg/m^3  DoExposeReferenceFrame=on  SerializedFrames=<Frames/>  GraphicType=FromGeometry  MarkerShape=Sphere  MarkerSize=10  GraphicVisPropType=SimpleVisualProperties  GraphicDiffuseColor=smiData.Solid(5).color  GraphicSpecularColor=[0.5 0.5 0.5 1.0]  GraphicAmbientColor=[0.15 0.15 0.15 1.0]  GraphicEmissiveColor=[0.0 0.0 0.0 1.0]  GraphicShininess=75  GraphicOpacity=smiData.Solid(5).opacity
  F : PMIOPort  Side=Left
  connections:
  Solid/RConn1 -- ReferenceFrame/RConn1 -- F/RConn1

== system EsamblajeCohete2_0/Cohete/Assembly_1_RIGID/Magnet_8_RIGID ==
  ReferenceFrame : sm_lib/Frames and Transforms/Reference Frame
  Solid : sm_lib/Body Elements/File Solid  ExtGeomFileName=Magnet_Default_sldprt.STEP  UnitType=FromFile  ExtGeomFileUnits=m  StepReaderType=HEX  ExportConvexHullGeometry=off  InertiaType=Custom  Mass=smiData.Solid(5).mass  MassUnits=kg  CenterOfMass=smiData.Solid(5).CoM  CenterOfMassUnits=mm  MomentsOfInertia=smiData.Solid(5).MoI  MomentsOfInertiaUnits=kg*mm^2  ProductsOfInertia=smiData.Solid(5).PoI  ProductsOfInertiaUnits=kg*mm^2  BasedOnType=DensityFromFile  Density=1000  DensityUnits=kg/m^3  DoExposeReferenceFrame=on  SerializedFrames=<Frames/>  GraphicType=FromGeometry  MarkerShape=Sphere  MarkerSize=10  GraphicVisPropType=SimpleVisualProperties  GraphicDiffuseColor=smiData.Solid(5).color  GraphicSpecularColor=[0.5 0.5 0.5 1.0]  GraphicAmbientColor=[0.15 0.15 0.15 1.0]  GraphicEmissiveColor=[0.0 0.0 0.0 1.0]  GraphicShininess=75  GraphicOpacity=smiData.Solid(5).opacity
  F : PMIOPort  Side=Left
  connections:
  Solid/RConn1 -- ReferenceFrame/RConn1 -- F/RConn1

== system EsamblajeCohete2_0/Cohete/Assembly_1_RIGID/Magnet_9_RIGID ==
  ReferenceFrame : sm_lib/Frames and Transforms/Reference Frame
  Solid : sm_lib/Body Elements/File Solid  ExtGeomFileName=Magnet_Default_sldprt.STEP  UnitType=FromFile  ExtGeomFileUnits=m  StepReaderType=HEX  ExportConvexHullGeometry=off  InertiaType=Custom  Mass=smiData.Solid(5).mass  MassUnits=kg  CenterOfMass=smiData.Solid(5).CoM  CenterOfMassUnits=mm  MomentsOfInertia=smiData.Solid(5).MoI  MomentsOfInertiaUnits=kg*mm^2  ProductsOfInertia=smiData.Solid(5).PoI  ProductsOfInertiaUnits=kg*mm^2  BasedOnType=DensityFromFile  Density=1000  DensityUnits=kg/m^3  DoExposeReferenceFrame=on  SerializedFrames=<Frames/>  GraphicType=FromGeometry  MarkerShape=Sphere  MarkerSize=10  GraphicVisPropType=SimpleVisualProperties  GraphicDiffuseColor=smiData.Solid(5).color  GraphicSpecularColor=[0.5 0.5 0.5 1.0]  GraphicAmbientColor=[0.15 0.15 0.15 1.0]  GraphicEmissiveColor=[0.0 0.0 0.0 1.0]  GraphicShininess=75  GraphicOpacity=smiData.Solid(5).opacity
  F : PMIOPort  Side=Left
  connections:
  Solid/RConn1 -- ReferenceFrame/RConn1 -- F/RConn1

== system EsamblajeCohete2_0/Cohete/Assembly_1_RIGID/Motor_Casing_1_RIGID ==
  ReferenceFrame : sm_lib/Frames and Transforms/Reference Frame
  Solid : sm_lib/Body Elements/File Solid  ExtGeomFileName=Motor Casing_Default_sldprt.STEP  UnitType=FromFile  ExtGeomFileUnits=m  StepReaderType=HEX  ExportConvexHullGeometry=off  InertiaType=Custom  Mass=smiData.Solid(8).mass  MassUnits=kg  CenterOfMass=smiData.Solid(8).CoM  CenterOfMassUnits=mm  MomentsOfInertia=smiData.Solid(8).MoI  MomentsOfInertiaUnits=kg*mm^2  ProductsOfInertia=smiData.Solid(8).PoI  ProductsOfInertiaUnits=kg*mm^2  BasedOnType=DensityFromFile  Density=1000  DensityUnits=kg/m^3  DoExposeReferenceFrame=on  SerializedFrames=<Frames/>  GraphicType=FromGeometry  MarkerShape=Sphere  MarkerSize=10  GraphicVisPropType=SimpleVisualProperties  GraphicDiffuseColor=smiData.Solid(8).color  GraphicSpecularColor=[0.5 0.5 0.5 1.0]  GraphicAmbientColor=[0.15 0.15 0.15 1.0]  GraphicEmissiveColor=[0.0 0.0 0.0 1.0]  GraphicShininess=75  GraphicOpacity=smiData.Solid(8).opacity
  F : PMIOPort  Side=Left
  connections:
  Solid/RConn1 -- ReferenceFrame/RConn1 -- F/RConn1

== system EsamblajeCohete2_0/Cohete/Assembly_1_RIGID/Nut_2_RIGID ==
  ReferenceFrame : sm_lib/Frames and Transforms/Reference Frame
  Solid : sm_lib/Body Elements/File Solid  ExtGeomFileName=Nut_Default_sldprt.STEP  UnitType=FromFile  ExtGeomFileUnits=m  StepReaderType=HEX  ExportConvexHullGeometry=off  InertiaType=Custom  Mass=smiData.Solid(13).mass  MassUnits=kg  CenterOfMass=smiData.Solid(13).CoM  CenterOfMassUnits=mm  MomentsOfInertia=smiData.Solid(13).MoI  MomentsOfInertiaUnits=kg*mm^2  ProductsOfInertia=smiData.Solid(13).PoI  ProductsOfInertiaUnits=kg*mm^2  BasedOnType=DensityFromFile  Density=1000  DensityUnits=kg/m^3  DoExposeReferenceFrame=on  SerializedFrames=<Frames/>  GraphicType=FromGeometry  MarkerShape=Sphere  MarkerSize=10  GraphicVisPropType=SimpleVisualProperties  GraphicDiffuseColor=smiData.Solid(13).color  GraphicSpecularColor=[0.5 0.5 0.5 1.0]  GraphicAmbientColor=[0.15 0.15 0.15 1.0]  GraphicEmissiveColor=[0.0 0.0 0.0 1.0]  GraphicShininess=75  GraphicOpacity=smiData.Solid(13).opacity
  F : PMIOPort  Side=Left
  connections:
  Solid/RConn1 -- ReferenceFrame/RConn1 -- F/RConn1

== system EsamblajeCohete2_0/Cohete/Assembly_1_RIGID/Rotor_1_RIGID ==
  ReferenceFrame : sm_lib/Frames and Transforms/Reference Frame
  Solid : sm_lib/Body Elements/File Solid  ExtGeomFileName=Rotor_Default_sldprt.STEP  UnitType=FromFile  ExtGeomFileUnits=m  StepReaderType=HEX  ExportConvexHullGeometry=off  InertiaType=Custom  Mass=smiData.Solid(9).mass  MassUnits=kg  CenterOfMass=smiData.Solid(9).CoM  CenterOfMassUnits=mm  MomentsOfInertia=smiData.Solid(9).MoI  MomentsOfInertiaUnits=kg*mm^2  ProductsOfInertia=smiData.Solid(9).PoI  ProductsOfInertiaUnits=kg*mm^2  BasedOnType=DensityFromFile  Density=1000  DensityUnits=kg/m^3  DoExposeReferenceFrame=on  SerializedFrames=<Frames/>  GraphicType=FromGeometry  MarkerShape=Sphere  MarkerSize=10  GraphicVisPropType=SimpleVisualProperties  GraphicDiffuseColor=smiData.Solid(9).color  GraphicSpecularColor=[0.5 0.5 0.5 1.0]  GraphicAmbientColor=[0.15 0.15 0.15 1.0]  GraphicEmissiveColor=[0.0 0.0 0.0 1.0]  GraphicShininess=75  GraphicOpacity=smiData.Solid(9).opacity
  F : PMIOPort  Side=Left
  connections:
  Solid/RConn1 -- ReferenceFrame/RConn1 -- F/RConn1

== system EsamblajeCohete2_0/Cohete/Assembly_1_RIGID/Rotor_Cover_1_RIGID ==
  ReferenceFrame : sm_lib/Frames and Transforms/Reference Frame
  Solid : sm_lib/Body Elements/File Solid  ExtGeomFileName=Rotor Cover_Default_sldprt.STEP  UnitType=FromFile  ExtGeomFileUnits=m  StepReaderType=HEX  ExportConvexHullGeometry=off  InertiaType=Custom  Mass=smiData.Solid(11).mass  MassUnits=kg  CenterOfMass=smiData.Solid(11).CoM  CenterOfMassUnits=mm  MomentsOfInertia=smiData.Solid(11).MoI  MomentsOfInertiaUnits=kg*mm^2  ProductsOfInertia=smiData.Solid(11).PoI  ProductsOfInertiaUnits=kg*mm^2  BasedOnType=DensityFromFile  Density=1000  DensityUnits=kg/m^3  DoExposeReferenceFrame=on  SerializedFrames=<Frames/>  GraphicType=FromGeometry  MarkerShape=Sphere  MarkerSize=10  GraphicVisPropType=SimpleVisualProperties  GraphicDiffuseColor=smiData.Solid(11).color  GraphicSpecularColor=[0.5 0.5 0.5 1.0]  GraphicAmbientColor=[0.15 0.15 0.15 1.0]  GraphicEmissiveColor=[0.0 0.0 0.0 1.0]  GraphicShininess=75  GraphicOpacity=smiData.Solid(11).opacity
  F : PMIOPort  Side=Left
  connections:
  Solid/RConn1 -- ReferenceFrame/RConn1 -- F/RConn1

== system EsamblajeCohete2_0/Cohete/Assembly_1_RIGID/Stopper_Screw_1_RIGID ==
  ReferenceFrame : sm_lib/Frames and Transforms/Reference Frame
  Solid : sm_lib/Body Elements/File Solid  ExtGeomFileName=Stopper Screw_Default_sldprt.STEP  UnitType=FromFile  ExtGeomFileUnits=m  StepReaderType=HEX  ExportConvexHullGeometry=off  InertiaType=Custom  Mass=smiData.Solid(12).mass  MassUnits=kg  CenterOfMass=smiData.Solid(12).CoM  CenterOfMassUnits=mm  MomentsOfInertia=smiData.Solid(12).MoI  MomentsOfInertiaUnits=kg*mm^2  ProductsOfInertia=smiData.Solid(12).PoI  ProductsOfInertiaUnits=kg*mm^2  BasedOnType=DensityFromFile  Density=1000  DensityUnits=kg/m^3  DoExposeReferenceFrame=on  SerializedFrames=<Frames/>  GraphicType=FromGeometry  MarkerShape=Sphere  MarkerSize=10  GraphicVisPropType=SimpleVisualProperties  GraphicDiffuseColor=smiData.Solid(12).color  GraphicSpecularColor=[0.5 0.5 0.5 1.0]  GraphicAmbientColor=[0.15 0.15 0.15 1.0]  GraphicEmissiveColor=[0.0 0.0 0.0 1.0]  GraphicShininess=75  GraphicOpacity=smiData.Solid(12).opacity
  F : PMIOPort  Side=Left
  connections:
  Solid/RConn1 -- ReferenceFrame/RConn1 -- F/RConn1

== system EsamblajeCohete2_0/Cohete/Assembly_1_RIGID/e_ring_external_retaining_ring_wti_4_RIGID ==
  ReferenceFrame : sm_lib/Frames and Transforms/Reference Frame
  Solid : sm_lib/Body Elements/File Solid  ExtGeomFileName=e-ring external retaining ring_wti_Truarc X5133-14 - S0.14_sldprt.STEP  UnitType=FromFile  ExtGeomFileUnits=m  StepReaderType=HEX  ExportConvexHullGeometry=off  InertiaType=Custom  Mass=smiData.Solid(10).mass  MassUnits=kg  CenterOfMass=smiData.Solid(10).CoM  CenterOfMassUnits=in  MomentsOfInertia=smiData.Solid(10).MoI  MomentsOfInertiaUnits=kg*in^2  ProductsOfInertia=smiData.Solid(10).PoI  ProductsOfInertiaUnits=kg*in^2  BasedOnType=DensityFromFile  Density=1000  DensityUnits=kg/m^3  DoExposeReferenceFrame=on  SerializedFrames=<Frames/>  GraphicType=FromGeometry  MarkerShape=Sphere  MarkerSize=10  GraphicVisPropType=SimpleVisualProperties  GraphicDiffuseColor=smiData.Solid(10).color  GraphicSpecularColor=[0.5 0.5 0.5 1.0]  GraphicAmbientColor=[0.15 0.15 0.15 1.0]  GraphicEmissiveColor=[0.0 0.0 0.0 1.0]  GraphicShininess=75  GraphicOpacity=smiData.Solid(10).opacity
  F : PMIOPort  Side=Left
  connections:
  Solid/RConn1 -- ReferenceFrame/RConn1 -- F/RConn1

== system EsamblajeCohete2_0/Cohete/Assembly_1_RIGID/instrument_ball_bearing_68_iso_1_RIGID ==
  ReferenceFrame : sm_lib/Frames and Transforms/Reference Frame
  Solid : sm_lib/Body Elements/File Solid  ExtGeomFileName=instrument ball bearing_68_iso_ISO 1224 - 390308 - R-8-DE-NC-8_68_sldprt.STEP  UnitType=FromFile  ExtGeomFileUnits=m  StepReaderType=HEX  ExportConvexHullGeometry=off  InertiaType=Custom  Mass=smiData.Solid(14).mass  MassUnits=kg  CenterOfMass=smiData.Solid(14).CoM  CenterOfMassUnits=mm  MomentsOfInertia=smiData.Solid(14).MoI  MomentsOfInertiaUnits=kg*mm^2  ProductsOfInertia=smiData.Solid(14).PoI  ProductsOfInertiaUnits=kg*mm^2  BasedOnType=DensityFromFile  Density=1000  DensityUnits=kg/m^3  DoExposeReferenceFrame=on  SerializedFrames=<Frames/>  GraphicType=FromGeometry  MarkerShape=Sphere  MarkerSize=10  GraphicVisPropType=SimpleVisualProperties  GraphicDiffuseColor=smiData.Solid(14).color  GraphicSpecularColor=[0.5 0.5 0.5 1.0]  GraphicAmbientColor=[0.15 0.15 0.15 1.0]  GraphicEmissiveColor=[0.0 0.0 0.0 1.0]  GraphicShininess=75  GraphicOpacity=smiData.Solid(14).opacity
  F : PMIOPort  Side=Left
  connections:
  Solid/RConn1 -- ReferenceFrame/RConn1 -- F/RConn1

== system EsamblajeCohete2_0/Cohete/Assembly_2_RIGID/Drive_Shaft_1_RIGID ==
  ReferenceFrame : sm_lib/Frames and Transforms/Reference Frame
  Solid : sm_lib/Body Elements/File Solid  ExtGeomFileName=Drive Shaft_Default_sldprt.STEP  UnitType=FromFile  ExtGeomFileUnits=m  StepReaderType=HEX  ExportConvexHullGeometry=off  InertiaType=Custom  Mass=smiData.Solid(7).mass  MassUnits=kg  CenterOfMass=smiData.Solid(7).CoM  CenterOfMassUnits=mm  MomentsOfInertia=smiData.Solid(7).MoI  MomentsOfInertiaUnits=kg*mm^2  ProductsOfInertia=smiData.Solid(7).PoI  ProductsOfInertiaUnits=kg*mm^2  BasedOnType=DensityFromFile  Density=1000  DensityUnits=kg/m^3  DoExposeReferenceFrame=on  SerializedFrames=<Frames/>  GraphicType=FromGeometry  MarkerShape=Sphere  MarkerSize=10  GraphicVisPropType=SimpleVisualProperties  GraphicDiffuseColor=smiData.Solid(7).color  GraphicSpecularColor=[0.5 0.5 0.5 1.0]  GraphicAmbientColor=[0.15 0.15 0.15 1.0]  GraphicEmissiveColor=[0.0 0.0 0.0 1.0]  GraphicShininess=75  GraphicOpacity=smiData.Solid(7).opacity
  F : PMIOPort  Side=Left
  connections:
  Solid/RConn1 -- ReferenceFrame/RConn1 -- F/RConn1
